simulink model "Test1_Non_exponential"  (R2014a)
settings: Solver=ode45  StartTime=0.0  StopTime=500  RelTol=1e-3
settings Model: Creator=KOO  LastModifiedBy=KOO

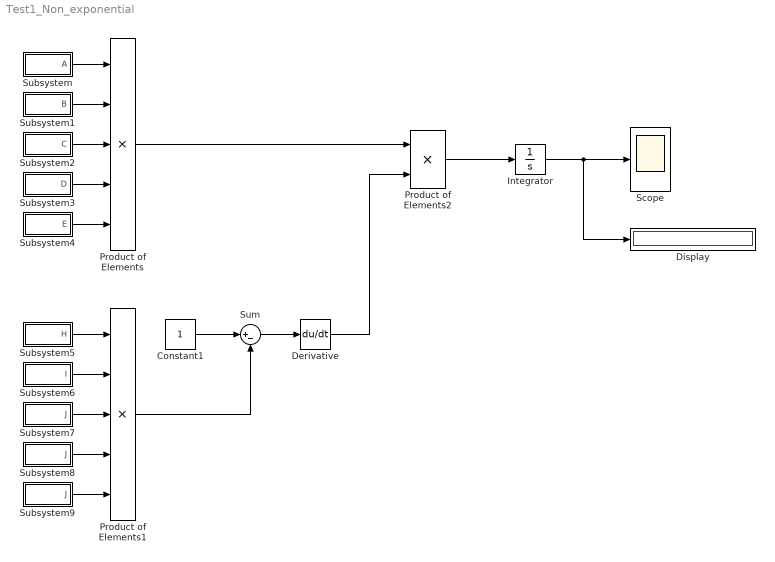
== system Test1_Non_exponential ==
  Constant1 : Constant
  Derivative : Derivative
  Display : Display
  Integrator : Integrator
  Product of Elements : Product  Inputs=5
  Product of Elements1 : Product  Inputs=5
  Product of Elements2 : Product
  Scope : Scope
      settings: YMin=0.95095  YMax=1.05105  SaveName=Merle_Out
  Subsystem : Subsystem
  Subsystem1 : Subsystem
  Subsystem2 : Subsystem
  Subsystem3 : Subsystem
  Subsystem4 : Subsystem
  Subsystem5 : Subsystem
  Subsystem6 : Subsystem
  Subsystem7 : Subsystem
  Subsystem8 : Subsystem
  Subsystem9 : Subsystem
  Sum : Sum  Inputs=|+-
  wires:
  Integrator/1 -> Scope/1, Display/1
  Subsystem/1(A) -> Product of Elements/1
  Subsystem1/1(B) -> Product of Elements/2
  Subsystem2/1("C ") -> Product of Elements/3
  Subsystem3/1(D) -> Product of Elements/4
  Subsystem4/1(E) -> Product of Elements/5
  Subsystem5/1(H) -> Product of Elements1/1
  Subsystem6/1(I) -> Product of Elements1/2
  Subsystem7/1(J) -> Product of Elements1/3
  Subsystem8/1(J) -> Product of Elements1/4
  Subsystem9/1(J) -> Product of Elements1/5
  Constant1/1 -> Sum/1
  Product of Elements1/1 -> Sum/2
  Sum/1 -> Derivative/1
  Product of Elements/1 -> Product of Elements2/1
  Derivative/1 -> Product of Elements2/2
  Product of Elements2/1 -> Integrator/1

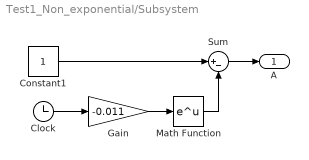
== system Test1_Non_exponential/Subsystem ==
  Clock : Clock
  Constant1 : Constant
  Gain : Gain  Gain=-0.011
  Math Function : Math  SaturateOnIntegerOverflow=on
  Sum : Sum  Inputs=|+-
  A : Outport
  wires:
  Constant1/1 -> Sum/1
  Math Function/1 -> Sum/2
  Sum/1 -> A/1
  Gain/1 -> Math Function/1
  Clock/1 -> Gain/1

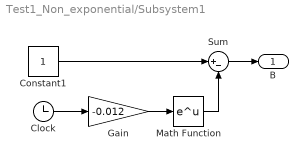
== system Test1_Non_exponential/Subsystem1 ==
  Clock : Clock
  Constant1 : Constant
  Gain : Gain  Gain=-0.012
  Math Function : Math  SaturateOnIntegerOverflow=on
  Sum : Sum  Inputs=|+-
  B : Outport
  wires:
  Clock/1 -> Gain/1
  Gain/1 -> Math Function/1
  Sum/1 -> B/1
  Math Function/1 -> Sum/2
  Constant1/1 -> Sum/1

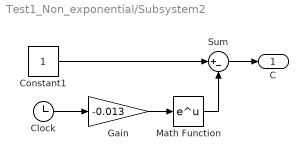
== system Test1_Non_exponential/Subsystem2 ==
  Clock : Clock
  Constant1 : Constant
  Gain : Gain  Gain=-0.013
  Math Function : Math  SaturateOnIntegerOverflow=on
  Sum : Sum  Inputs=|+-
  "C " : Outport
  wires:
  Constant1/1 -> Sum/1
  Math Function/1 -> Sum/2
  Sum/1 -> "C "/1
  Gain/1 -> Math Function/1
  Clock/1 -> Gain/1

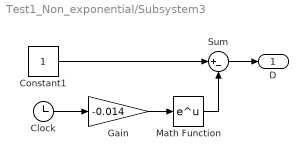
== system Test1_Non_exponential/Subsystem3 ==
  Clock : Clock
  Constant1 : Constant
  Gain : Gain  Gain=-0.014
  Math Function : Math  SaturateOnIntegerOverflow=on
  Sum : Sum  Inputs=|+-
  D : Outport
  wires:
  Clock/1 -> Gain/1
  Gain/1 -> Math Function/1
  Sum/1 -> D/1
  Math Function/1 -> Sum/2
  Constant1/1 -> Sum/1

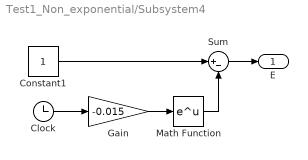
== system Test1_Non_exponential/Subsystem4 ==
  Clock : Clock
  Constant1 : Constant
  Gain : Gain  Gain=-0.015
  Math Function : Math  SaturateOnIntegerOverflow=on
  Sum : Sum  Inputs=|+-
  E : Outport
  wires:
  Constant1/1 -> Sum/1
  Math Function/1 -> Sum/2
  Sum/1 -> E/1
  Gain/1 -> Math Function/1
  Clock/1 -> Gain/1

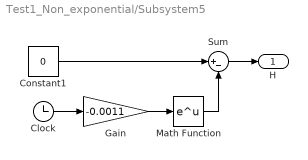
== system Test1_Non_exponential/Subsystem5 ==
  Clock : Clock
  Constant1 : Constant  Value=0
  Gain : Gain  Gain=-0.0011
  Math Function : Math  SaturateOnIntegerOverflow=on
  Sum : Sum  Inputs=|+-
  H : Outport
  wires:
  Clock/1 -> Gain/1
  Gain/1 -> Math Function/1
  Sum/1 -> H/1
  Math Function/1 -> Sum/2
  Constant1/1 -> Sum/1

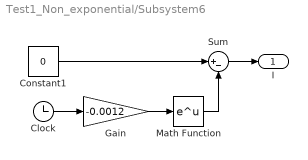
== system Test1_Non_exponential/Subsystem6 ==
  Clock : Clock
  Constant1 : Constant  Value=0
  Gain : Gain  Gain=-0.0012
  Math Function : Math  SaturateOnIntegerOverflow=on
  Sum : Sum  Inputs=|+-
  I : Outport
  wires:
  Constant1/1 -> Sum/1
  Math Function/1 -> Sum/2
  Sum/1 -> I/1
  Gain/1 -> Math Function/1
  Clock/1 -> Gain/1

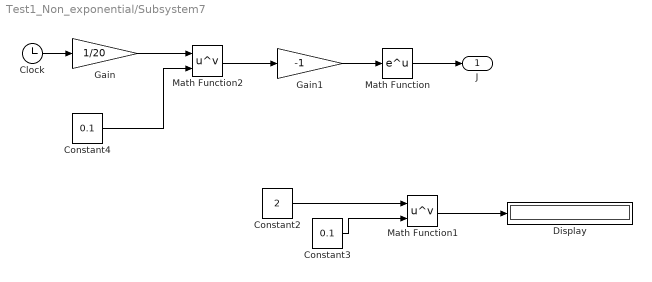
== system Test1_Non_exponential/Subsystem7 ==
  Clock : Clock
  Constant2 : Constant  Value=2
  Constant3 : Constant  Value=0.1
  Constant4 : Constant  Value=0.1
  Display : Display
  Gain : Gain  Gain=1/20
  Gain1 : Gain  Gain=-1
  Math Function : Math  SaturateOnIntegerOverflow=on
  Math Function1 : Math  Operator=pow  SaturateOnIntegerOverflow=on
  Math Function2 : Math  Operator=pow  SaturateOnIntegerOverflow=on
  J : Outport
  wires:
  Clock/1 -> Gain/1
  Math Function/1 -> J/1
  Constant2/1 -> Math Function1/1
  Constant3/1 -> Math Function1/2
  Math Function1/1 -> Display/1
  Gain/1 -> Math Function2/1
  Constant4/1 -> Math Function2/2
  Math Function2/1 -> Gain1/1
  Gain1/1 -> Math Function/1

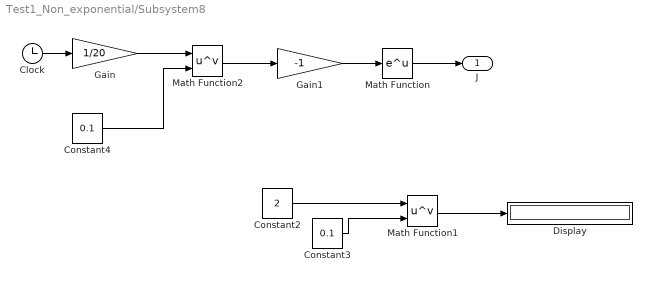
== system Test1_Non_exponential/Subsystem8 ==
  Clock : Clock
  Constant2 : Constant  Value=2
  Constant3 : Constant  Value=0.1
  Constant4 : Constant  Value=0.1
  Display : Display
  Gain : Gain  Gain=1/20
  Gain1 : Gain  Gain=-1
  Math Function : Math  SaturateOnIntegerOverflow=on
  Math Function1 : Math  Operator=pow  SaturateOnIntegerOverflow=on
  Math Function2 : Math  Operator=pow  SaturateOnIntegerOverflow=on
  J : Outport
  wires:
  Gain1/1 -> Math Function/1
  Math Function2/1 -> Gain1/1
  Constant4/1 -> Math Function2/2
  Gain/1 -> Math Function2/1
  Math Function1/1 -> Display/1
  Constant3/1 -> Math Function1/2
  Constant2/1 -> Math Function1/1
  Math Function/1 -> J/1
  Clock/1 -> Gain/1

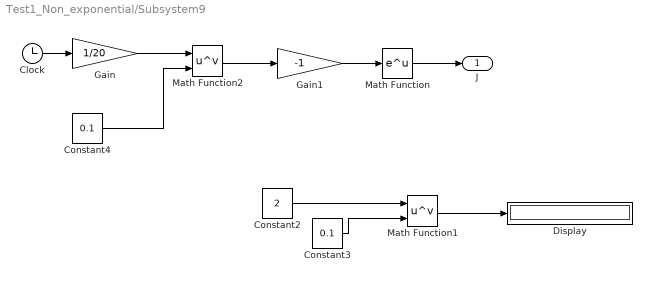
== system Test1_Non_exponential/Subsystem9 ==
  Clock : Clock
  Constant2 : Constant  Value=2
  Constant3 : Constant  Value=0.1
  Constant4 : Constant  Value=0.1
  Display : Display
  Gain : Gain  Gain=1/20
  Gain1 : Gain  Gain=-1
  Math Function : Math  SaturateOnIntegerOverflow=on
  Math Function1 : Math  Operator=pow  SaturateOnIntegerOverflow=on
  Math Function2 : Math  Operator=pow  SaturateOnIntegerOverflow=on
  J : Outport
  wires:
  Clock/1 -> Gain/1
  Math Function/1 -> J/1
  Constant2/1 -> Math Function1/1
  Constant3/1 -> Math Function1/2
  Math Function1/1 -> Display/1
  Gain/1 -> Math Function2/1
  Constant4/1 -> Math Function2/2
  Math Function2/1 -> Gain1/1
  Gain1/1 -> Math Function/1
